simulink library "neural"  (R2016b)
settings: Solver=ode45  StartTime=0.0  StopTime=10.0  RelTol=1e-3
undefined symbols (not defined in the file): sfunxy2
libraries: simulink x2
(part 2 of 2)

== system neural/Transfer Functions/elliotsig ==
  n : Inport
  Abs : Abs
  Divide : Product  Inputs=*/
  Sum : Sum  SaturateOnIntegerOverflow=on  InputSameDT=on  OutDataTypeStr=Inherit: Same as first input
  one : Constant
  a : Outport  InitialOutput=0
  wires:
  Sum/1 -> Divide/2
  Divide/1 -> a/1
  Abs/1 -> Sum/1
  n/1 -> Divide/1, Abs/1
  one/1 -> Sum/2

== system neural/Transfer Functions/hardlim ==
  n : Inport
  Constant : Constant
  Constant1 : Constant  Value=0
  Switch : Switch
  a : Outport  InitialOutput=0
  wires:
  Switch/1 -> a/1
  n/1 -> Switch/2
  Constant1/1 -> Switch/3
  Constant/1 -> Switch/1

== system neural/Transfer Functions/hardlims ==
  n : Inport
  Constant : Constant
  Constant1 : Constant  Value=-1
  Switch : Switch
  a : Outport  InitialOutput=0
  wires:
  Switch/1 -> a/1
  n/1 -> Switch/2
  Constant1/1 -> Switch/3
  Constant/1 -> Switch/1

== system neural/Transfer Functions/logsig ==
  n : Inport
  Exp : Math  SaturateOnIntegerOverflow=on
  Gain : Gain  Gain=-1  SaturateOnIntegerOverflow=on  OutDataTypeStr=Inherit: Same as input  ParamDataTypeStr=Inherit: Same as input
  Reciprocal : Math  Operator=reciprocal  SaturateOnIntegerOverflow=on
  Sum : Sum  SaturateOnIntegerOverflow=on  InputSameDT=on  OutDataTypeStr=Inherit: Same as first input
  one : Constant
  a : Outport  InitialOutput=0
  wires:
  Reciprocal/1 -> a/1
  Sum/1 -> Reciprocal/1
  one/1 -> Sum/2
  Exp/1 -> Sum/1
  Gain/1 -> Exp/1
  n/1 -> Gain/1

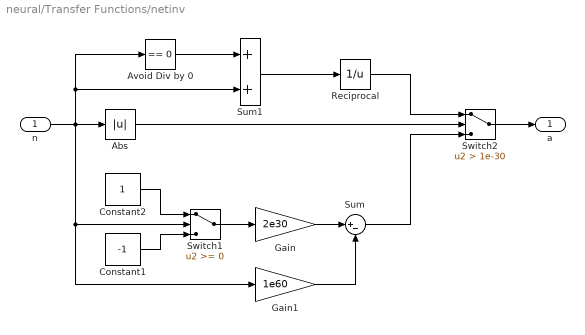
== system neural/Transfer Functions/netinv ==
  n : Inport
  Abs : Abs
  Avoid Div by 0 : simulink/Logic and Bit Operations/Compare To Constant  relop===  const=0  OutDataTypeStr=uint8
  Constant1 : Constant  Value=-1
  Constant2 : Constant
  Gain : Gain  Gain=2e30
  Gain1 : Gain  Gain=1e60
  Reciprocal : Math  Operator=reciprocal  SaturateOnIntegerOverflow=on
  Sum : Sum  Inputs=|+-
  Sum1 : Sum
  Switch1 : Switch
  Switch2 : Switch  Criteria=u2 > Threshold  Threshold=1e-30
  a : Outport  InitialOutput=0
  wires:
  n/1 -> Abs/1, Gain1/1, Switch1/2, Avoid Div by 0/1, Sum1/2
  Abs/1 -> Switch2/2
  Gain/1 -> Sum/1
  Gain1/1 -> Sum/2
  Sum/1 -> Switch2/3
  Constant1/1 -> Switch1/3
  Constant2/1 -> Switch1/1
  Switch1/1 -> Gain/1
  Switch2/1 -> a/1
  Avoid Div by 0/1 -> Sum1/1
  Sum1/1 -> Reciprocal/1
  Reciprocal/1 -> Switch2/1

== system neural/Transfer Functions/poslin ==
  n : Inport
  Saturation : Saturate  UpperLimit=inf  LowerLimit=0
  a : Outport  InitialOutput=0
  wires:
  n/1 -> Saturation/1
  Saturation/1 -> a/1

== system neural/Transfer Functions/purelin ==
  n : Inport
  a : Outport  InitialOutput=0
  wires:
  n/1 -> a/1

== system neural/Transfer Functions/radbas ==
  n : Inport
  Exp : Math  SaturateOnIntegerOverflow=on
  Gain : Gain  Gain=-1  SaturateOnIntegerOverflow=on  OutDataTypeStr=Inherit: Same as input  ParamDataTypeStr=Inherit: Same as input
  Product : Product  SaturateOnIntegerOverflow=on  RndMeth=Zero  InputSameDT=on  OutDataTypeStr=Inherit: Same as first input
  a : Outport  InitialOutput=0
  wires:
  Exp/1 -> a/1
  Gain/1 -> Exp/1
  Product/1 -> Gain/1
  n/1 -> Product/2, Product/1

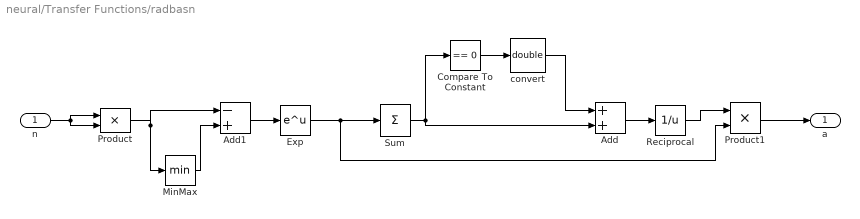
== system neural/Transfer Functions/radbasn ==
  n : Inport
  Add : Sum
  Add1 : Sum  Inputs=-+
  Compare To Constant : simulink/Logic and Bit Operations/Compare To Constant  relop===  const=0  OutDataTypeStr=uint8
  Exp : Math  SaturateOnIntegerOverflow=on
  MinMax : MinMax
  Product : Product  SaturateOnIntegerOverflow=on  RndMeth=Zero  InputSameDT=on  OutDataTypeStr=Inherit: Same as first input
  Product1 : Product  SaturateOnIntegerOverflow=on  RndMeth=Zero  InputSameDT=on  OutDataTypeStr=Inherit: Same as first input
  Reciprocal : Math  Operator=reciprocal  SaturateOnIntegerOverflow=on
  Sum : Sum  Inputs=+  SaturateOnIntegerOverflow=on  InputSameDT=on  OutDataTypeStr=Inherit: Same as first input
  convert : DataTypeConversion  OutDataTypeStr=double
  a : Outport  InitialOutput=0
  wires:
  n/1 -> Product/1, Product/2
  Product/1 -> MinMax/1, Add1/1
  Add1/1 -> Exp/1
  Sum/1 -> Compare To Constant/1, Add/2
  Product1/1 -> a/1
  Reciprocal/1 -> Product1/1
  Exp/1 -> Sum/1, Product1/2
  Compare To Constant/1 -> convert/1
  Add/1 -> Reciprocal/1
  convert/1 -> Add/1
  MinMax/1 -> Add1/2

== system neural/Transfer Functions/satlin ==
  n : Inport
  Saturation : Saturate  UpperLimit=1  LowerLimit=0
  a : Outport  InitialOutput=0
  wires:
  n/1 -> Saturation/1
  Saturation/1 -> a/1

== system neural/Transfer Functions/satlins ==
  n : Inport
  Saturation : Saturate  UpperLimit=1  LowerLimit=-1
  a : Outport  InitialOutput=0
  wires:
  n/1 -> Saturation/1
  Saturation/1 -> a/1

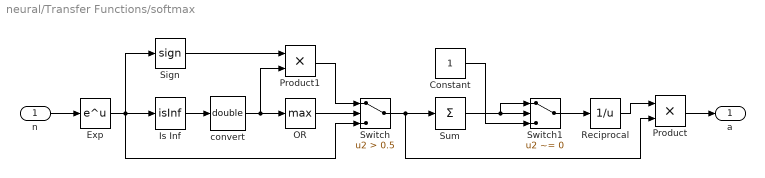
== system neural/Transfer Functions/softmax ==
  n : Inport
  Constant : Constant
  Exp : Math  SaturateOnIntegerOverflow=on
  Is Inf : RelationalOperator  Operator=isInf  OutDataTypeStr=fixdt(1,16)  RndMeth=Nearest
  OR : MinMax  Function=max
  Product : Product  SaturateOnIntegerOverflow=on  RndMeth=Zero  InputSameDT=on  OutDataTypeStr=Inherit: Same as first input
  Product1 : Product  SaturateOnIntegerOverflow=on  RndMeth=Zero  InputSameDT=on  OutDataTypeStr=Inherit: Same as first input
  Reciprocal : Math  Operator=reciprocal  SaturateOnIntegerOverflow=on
  Sign : Signum
  Sum : Sum  Inputs=+  SaturateOnIntegerOverflow=on  InputSameDT=on  OutDataTypeStr=Inherit: Same as first input
  Switch : Switch  Criteria=u2 > Threshold  Threshold=0.5
  Switch1 : Switch  Criteria=u2 ~= 0  Threshold=0.5
  convert : DataTypeConversion  OutDataTypeStr=double
  a : Outport  InitialOutput=0
  wires:
  Product/1 -> a/1
  n/1 -> Exp/1
  Is Inf/1 -> convert/1
  convert/1 -> OR/1, Product1/2
  Switch/1 -> Sum/1, Product/2
  OR/1 -> Switch/2
  Exp/1 -> Switch/3, Sign/1, Is Inf/1
  Sign/1 -> Product1/1
  Product1/1 -> Switch/1
  Switch1/1 -> Reciprocal/1
  Reciprocal/1 -> Product/1
  Sum/1 -> Switch1/2, Switch1/1
  Constant/1 -> Switch1/3

== system neural/Transfer Functions/tansig ==
  n : Inport
  Exp : Math  SaturateOnIntegerOverflow=on
  Gain : Gain  Gain=-2  SaturateOnIntegerOverflow=on  OutDataTypeStr=Inherit: Same as input  ParamDataTypeStr=Inherit: Same as input
  Gain1 : Gain  Gain=2  SaturateOnIntegerOverflow=on  OutDataTypeStr=Inherit: Same as input  ParamDataTypeStr=Inherit: Same as input
  Reciprocal : Math  Operator=reciprocal  SaturateOnIntegerOverflow=on
  Sum : Sum  SaturateOnIntegerOverflow=on  InputSameDT=on  OutDataTypeStr=Inherit: Same as first input
  Sum1 : Sum  Inputs=+-  SaturateOnIntegerOverflow=on  InputSameDT=on  OutDataTypeStr=Inherit: Same as first input
  one : Constant
  one1 : Constant
  a : Outport  InitialOutput=0
  wires:
  Sum1/1 -> a/1
  one1/1 -> Sum1/2
  Gain1/1 -> Sum1/1
  Reciprocal/1 -> Gain1/1
  Sum/1 -> Reciprocal/1
  one/1 -> Sum/2
  Exp/1 -> Sum/1
  Gain/1 -> Exp/1
  n/1 -> Gain/1

== system neural/Transfer Functions/tribas ==
  In1 : Inport
  Abs : Abs  SaturateOnIntegerOverflow=on
  MinMax : MinMax  Function=max  Inputs=2  SaturateOnIntegerOverflow=on  InputSameDT=on
  Sum : Sum  Inputs=+-  SaturateOnIntegerOverflow=on  InputSameDT=on  OutDataTypeStr=Inherit: Same as first input
  one : Constant
  zero : Constant  Value=0
  Out1 : Outport  InitialOutput=0
  wires:
  one/1 -> Sum/1
  In1/1 -> Abs/1
  Abs/1 -> Sum/2
  Sum/1 -> MinMax/1
  zero/1 -> MinMax/2
  MinMax/1 -> Out1/1

== system neural/Weight Functions/dist ==
  w : Inport
  p : Inport  Port=2
  Diff : Sum  Inputs=+-  SaturateOnIntegerOverflow=on  InputSameDT=on  OutDataTypeStr=Inherit: Same as first input
  Product : Product  SaturateOnIntegerOverflow=on  RndMeth=Zero  InputSameDT=on  OutDataTypeStr=Inherit: Same as first input
  Sqrt : Math  Operator=sqrt  SaturateOnIntegerOverflow=on
  Sum : Sum  Inputs=1  SaturateOnIntegerOverflow=on  InputSameDT=on  OutDataTypeStr=Inherit: Same as first input
  z : Outport  InitialOutput=0
  wires:
  Sqrt/1 -> z/1
  Sum/1 -> Sqrt/1
  Product/1 -> Sum/1
  Diff/1 -> Product/2, Product/1
  p/1 -> Diff/2
  w/1 -> Diff/1

== system neural/Weight Functions/dotprod ==
  In1 : Inport
  In2 : Inport  Port=2
  Dot Product : DotProduct  InputSameDT=on  OutDataTypeStr=Inherit: Inherit via internal rule
  Out1 : Outport
  wires:
  In1/1 -> Dot Product/1
  In2/1 -> Dot Product/2
  Dot Product/1 -> Out1/1

== system neural/Weight Functions/negdist ==
  w : Inport
  p : Inport  Port=2
  Diff : Sum  Inputs=+-  SaturateOnIntegerOverflow=on  InputSameDT=on  OutDataTypeStr=Inherit: Same as first input
  Gain : Gain  Gain=-1  SaturateOnIntegerOverflow=on  OutDataTypeStr=Inherit: Same as input  ParamDataTypeStr=Inherit: Same as input
  Product : Product  SaturateOnIntegerOverflow=on  RndMeth=Zero  InputSameDT=on  OutDataTypeStr=Inherit: Same as first input
  Sqrt : Math  Operator=sqrt  SaturateOnIntegerOverflow=on
  Sum : Sum  Inputs=1  SaturateOnIntegerOverflow=on  InputSameDT=on  OutDataTypeStr=Inherit: Same as first input
  z : Outport  InitialOutput=0
  wires:
  Gain/1 -> z/1
  Sqrt/1 -> Gain/1
  Sum/1 -> Sqrt/1
  Product/1 -> Sum/1
  Diff/1 -> Product/2, Product/1
  p/1 -> Diff/2
  w/1 -> Diff/1

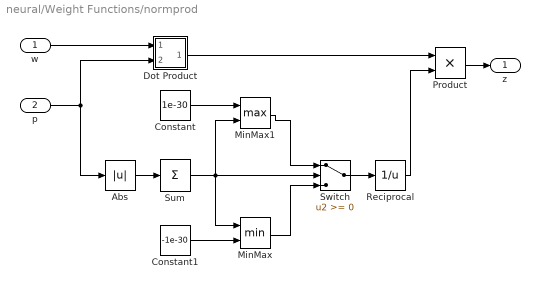
== system neural/Weight Functions/normprod ==
  w : Inport
  p : Inport  Port=2
  Abs : Abs
  Constant : Constant  Value=1e-30
  Constant1 : Constant  Value=-1e-30
  Dot Product : Subsystem  mask(Dot Product){}
      mask help:
      | Inner (dot) product.
      | y=sum(u1.*u2)
      mask init:
      | t=(0:.1:2*pi)';
      | x=cos(t);
      | y=sin(t);
      mask Help: Computes the inner (dot) product of the inputs: sum(u1.*u2).  The inputs are vectors of the same length. Output is a scalar.
      mask Display: plot(0,0,1,1,x*[0.025 0.07]+0.5,y*[0.025 0.07]+0.5)
  MinMax : MinMax  Inputs=2
  MinMax1 : MinMax  Function=max  Inputs=2
  Product : Product  SaturateOnIntegerOverflow=on  RndMeth=Zero  InputSameDT=on  OutDataTypeStr=Inherit: Same as first input
  Reciprocal : Math  Operator=reciprocal  SaturateOnIntegerOverflow=on
  Sum : Sum  Inputs=1  SaturateOnIntegerOverflow=on  InputSameDT=on  OutDataTypeStr=Inherit: Same as first input
  Switch : Switch
  z : Outport  InitialOutput=0
  wires:
  Product/1 -> z/1
  Dot Product/1(out_1) -> Product/1
  p/1 -> Dot Product/2(in_2), Abs/1
  w/1 -> Dot Product/1(in_1)
  Reciprocal/1 -> Product/2
  Sum/1 -> MinMax/1, MinMax1/2, Switch/2
  Constant/1 -> MinMax1/1
  Constant1/1 -> MinMax/2
  MinMax/1 -> Switch/3
  MinMax1/1 -> Switch/1
  Switch/1 -> Reciprocal/1
  Abs/1 -> Sum/1

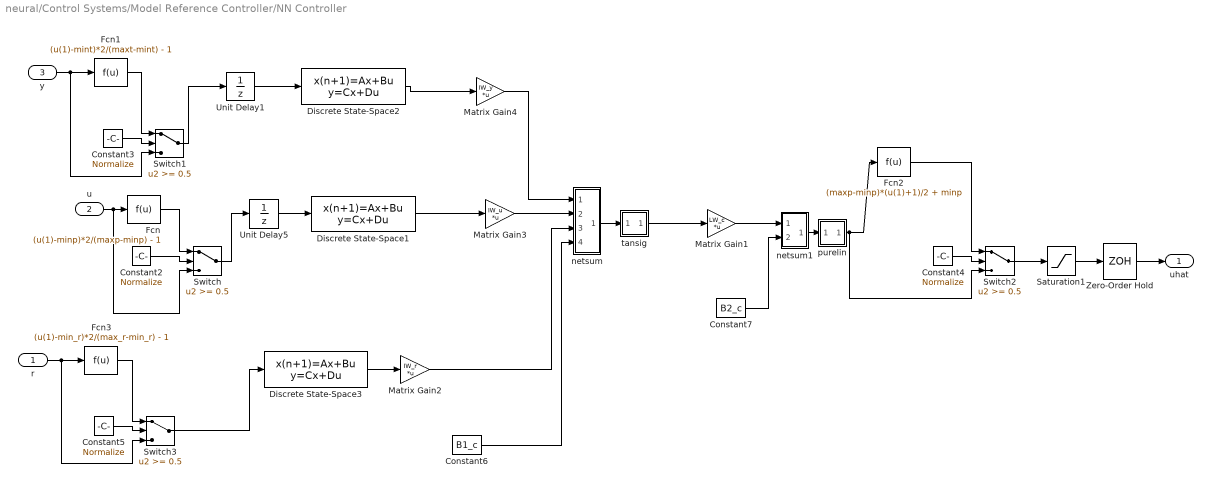
== system neural/Control Systems/Model Reference Controller/NN Controller ==
  r : Inport
  u : Inport  Port=2
  y : Inport  Port=3
  Constant{2..5} (4 alike) : Constant  Value=Normalize
  Constant6 : Constant  Value=B1_c
  Constant7 : Constant  Value=B2_c
  Discrete State-Space1 : DiscreteStateSpace  A=[zeros(1,max([Nic-1 1]));eye(Nic-2,Nic-1)]  B=eye(max([Nic-1 1]),1)  C=[zeros(1,max([Nic-1 1]));eye(Nic-1,Nic-1)]  D=eye(Nic,1)  SampleTime=Ts
  Discrete State-Space2 : DiscreteStateSpace  A=[zeros(1,max([Njc-1 1]));eye(Njc-2,Njc-1)]  B=eye(max([Njc-1 1]),1)  C=[zeros(1,max([Njc-1 1]));eye(Njc-1,Njc-1)]  D=eye(Njc,1)  SampleTime=Ts
  Discrete State-Space3 : DiscreteStateSpace  A=[zeros(1,max([Nrc-1 1]));eye(Nrc-2,Nrc-1)]  B=eye(max([Nrc-1 1]),1)  C=[zeros(1,max([Nrc-1 1]));eye(Nrc-1,Nrc-1)]  D=eye(Nrc,1)  SampleTime=Ts
  Fcn : Fcn  Expr=(u(1)-minp)*2/(maxp-minp) - 1
  Fcn1 : Fcn  Expr=(u(1)-mint)*2/(maxt-mint) - 1
  Fcn2 : Fcn  Expr=(maxp-minp)*(u(1)+1)/2 + minp
  Fcn3 : Fcn  Expr=(u(1)-min_r)*2/(max_r-min_r) - 1
  Matrix Gain1 : Gain  Gain=LW_c  Multiplication=Matrix(K*u)  SaturateOnIntegerOverflow=on  OutDataTypeStr=Inherit: Same as input  ParamDataTypeStr=Inherit: Same as input
  Matrix Gain2 : Gain  Gain=IW_r  Multiplication=Matrix(K*u)  SaturateOnIntegerOverflow=on  OutDataTypeStr=Inherit: Same as input  ParamDataTypeStr=Inherit: Same as input
  Matrix Gain3 : Gain  Gain=IW_u  Multiplication=Matrix(K*u)  SaturateOnIntegerOverflow=on  OutDataTypeStr=Inherit: Same as input  ParamDataTypeStr=Inherit: Same as input
  Matrix Gain4 : Gain  Gain=IW_y  Multiplication=Matrix(K*u)  SaturateOnIntegerOverflow=on  OutDataTypeStr=Inherit: Same as input  ParamDataTypeStr=Inherit: Same as input
  Saturation1 : Saturate  UpperLimit=max_i  LowerLimit=min_i
  Switch{,1..3} (4 alike) : Switch  Threshold=0.5  SaturateOnIntegerOverflow=on  InputSameDT=on
  Unit Delay1 : UnitDelay  SampleTime=Ts
  Unit Delay5 : UnitDelay  SampleTime=Ts
  Zero-Order Hold : ZeroOrderHold  SampleTime=Ts
  netsum : Subsystem
      mask Display: disp('+')
  netsum1 : Subsystem
      mask Display: disp('+')
  purelin : Subsystem
      mask Display: plot([-1 1],[0 0],[-1 1],[-1 1])
  tansig : Subsystem
      mask Display: plot([-1 1],[0 0],[-1 -.9 -.8 -.7 -.6 -.5 -.4 -.3 -.2 -.1 0 .1 .2 .3 .4 .5 .6 .7 .8 .9 1],2./(1+exp(-8*[-1 -.9 -.8 -.7 -.6 -.5 -.4 -.3 -.2 -.1 0 .1 .2 .3 .4 .5 .6 .7 .8 .9 1]))-1)
  uhat : Outport
  wires:
  Fcn2/1 -> Switch2/1
  Fcn/1 -> Switch/1
  Discrete State-Space1/1 -> Matrix Gain3/1
  tansig/1(a) -> Matrix Gain1/1
  Discrete State-Space2/1 -> Matrix Gain4/1
  Switch3/1 -> Discrete State-Space3/1
  Unit Delay1/1 -> Discrete State-Space2/1
  Unit Delay5/1 -> Discrete State-Space1/1
  Saturation1/1 -> Zero-Order Hold/1
  Zero-Order Hold/1 -> uhat/1
  Discrete State-Space3/1 -> Matrix Gain2/1
  Constant7/1 -> netsum1/2(In2)
  Switch2/1 -> Saturation1/1
  purelin/1(a) -> Fcn2/1, Switch2/3
  Constant4/1 -> Switch2/2
  Matrix Gain1/1 -> netsum1/1(In1)
  netsum1/1(Out1) -> purelin/1(n)
  Matrix Gain2/1 -> netsum/3(In3)
  netsum/1(Out1) -> tansig/1(n)
  r/1 -> Switch3/3, Fcn3/1
  Fcn3/1 -> Switch3/1
  Constant5/1 -> Switch3/2
  y/1 -> Switch1/3, Fcn1/1
  Fcn1/1 -> Switch1/1
  Switch1/1 -> Unit Delay1/1
  Constant3/1 -> Switch1/2
  Constant2/1 -> Switch/2
  u/1 -> Fcn/1, Switch/3
  Switch/1 -> Unit Delay5/1
  Constant6/1 -> netsum/4(In4)
  Matrix Gain3/1 -> netsum/2(In2)
  Matrix Gain4/1 -> netsum/1(In1)

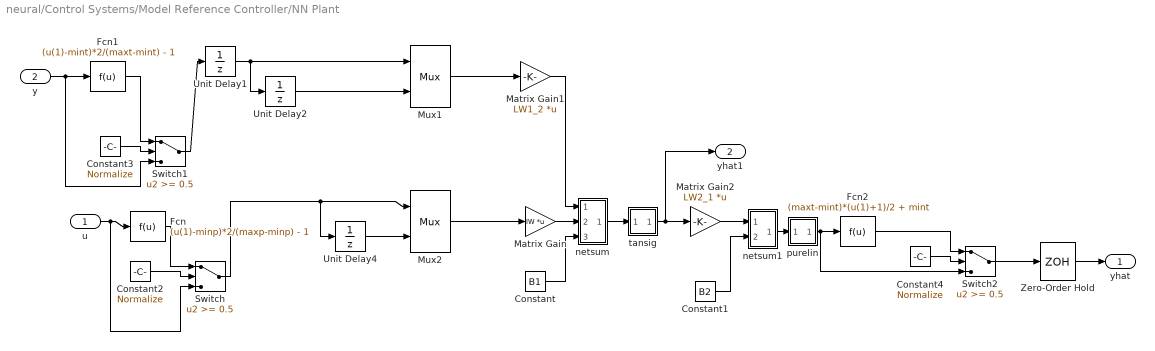
== system neural/Control Systems/Model Reference Controller/NN Plant ==
  u : Inport
  y : Inport  Port=2
  Constant : Constant  Value=B1
  Constant1 : Constant  Value=B2
  Constant2 : Constant  Value=Normalize
  Constant3 : Constant  Value=Normalize
  Constant4 : Constant  Value=Normalize
  Fcn : Fcn  Expr=(u(1)-minp)*2/(maxp-minp) - 1
  Fcn1 : Fcn  Expr=(u(1)-mint)*2/(maxt-mint) - 1
  Fcn2 : Fcn  Expr=(maxt-mint)*(u(1)+1)/2 + mint
  Matrix Gain : Gain  Gain=IW  Multiplication=Matrix(K*u)  SaturateOnIntegerOverflow=on  OutDataTypeStr=Inherit: Same as input  ParamDataTypeStr=Inherit: Same as input
  Matrix Gain1 : Gain  Gain=LW1_2  Multiplication=Matrix(K*u)  SaturateOnIntegerOverflow=on  OutDataTypeStr=Inherit: Same as input  ParamDataTypeStr=Inherit: Same as input
  Matrix Gain2 : Gain  Gain=LW2_1  Multiplication=Matrix(K*u)  SaturateOnIntegerOverflow=on  OutDataTypeStr=Inherit: Same as input  ParamDataTypeStr=Inherit: Same as input
  Mux1 : Mux  Inputs=2
      settings: DisplayOption=signals
  Mux2 : Mux  Inputs=2
      settings: DisplayOption=signals
  Switch : Switch  Threshold=0.5  SaturateOnIntegerOverflow=on  InputSameDT=on
  Switch1 : Switch  Threshold=0.5  SaturateOnIntegerOverflow=on  InputSameDT=on
  Switch2 : Switch  Threshold=0.5  SaturateOnIntegerOverflow=on  InputSameDT=on
  Unit Delay1 : UnitDelay  SampleTime=Ts
  Unit Delay2 : UnitDelay  SampleTime=Ts
  Unit Delay4 : UnitDelay  SampleTime=Ts
  Zero-Order Hold : ZeroOrderHold  SampleTime=Ts
  netsum : Subsystem
      mask Display: disp('+')
  netsum1 : Subsystem
      mask Display: disp('+')
  purelin : Subsystem
      mask Display: plot([-1 1],[0 0],[-1 1],[-1 1])
  tansig : Subsystem
      mask Display: plot([-1 1],[0 0],[-1 -.9 -.8 -.7 -.6 -.5 -.4 -.3 -.2 -.1 0 .1 .2 .3 .4 .5 .6 .7 .8 .9 1],2./(1+exp(-8*[-1 -.9 -.8 -.7 -.6 -.5 -.4 -.3 -.2 -.1 0 .1 .2 .3 .4 .5 .6 .7 .8 .9 1]))-1)
  yhat : Outport
  yhat1 : Outport  Port=2
  wires:
  Switch2/1 -> Zero-Order Hold/1
  Zero-Order Hold/1 -> yhat/1
  Switch/1 -> Unit Delay4/1, Mux2/1
  Unit Delay4/1 -> Mux2/2
  Unit Delay2/1 -> Mux1/2
  Unit Delay1/1 -> Unit Delay2/1, Mux1/1
  y/1 -> Switch1/3, Fcn1/1
  Fcn1/1 -> Switch1/1
  Switch1/1 -> Unit Delay1/1
  Constant3/1 -> Switch1/2
  Mux1/1 -> Matrix Gain1/1
  Constant2/1 -> Switch/2
  u/1 -> Switch/3, Fcn/1
  Fcn/1 -> Switch/1
  Mux2/1 -> Matrix Gain/1
  purelin/1(a) -> Switch2/3, Fcn2/1
  Fcn2/1 -> Switch2/1
  Constant4/1 -> Switch2/2
  tansig/1(a) -> yhat1/1, Matrix Gain2/1
  Matrix Gain/1 -> netsum/2(In2)
  Matrix Gain1/1 -> netsum/1(In1)
  Constant/1 -> netsum/3(In3)
  netsum/1(Out1) -> tansig/1(n)
  Matrix Gain2/1 -> netsum1/1(In1)
  Constant1/1 -> netsum1/2(In2)
  netsum1/1(Out1) -> purelin/1(n)

== system neural/Control Systems/NARMA-L2 Controller/netsum ==
  In1 : Inport
  In2 : Inport  Port=2
  netsum : Sum  Inputs=2  SaturateOnIntegerOverflow=on  InputSameDT=on  OutDataTypeStr=Inherit: Same as first input
  Out1 : Outport
  wires:
  netsum/1 -> Out1/1
  In2/1 -> netsum/2
  In1/1 -> netsum/1

== system neural/Control Systems/NARMA-L2 Controller/netsum1 ==
  In1 : Inport
  In2 : Inport  Port=2
  netsum1 : Sum  Inputs=2  SaturateOnIntegerOverflow=on  InputSameDT=on  OutDataTypeStr=Inherit: Same as first input
  Out1 : Outport
  wires:
  netsum1/1 -> Out1/1
  In2/1 -> netsum1/2
  In1/1 -> netsum1/1

== system neural/Control Systems/NARMA-L2 Controller/netsum2 ==
  In1 : Inport
  In2 : Inport  Port=2
  netsum : Sum  Inputs=2  SaturateOnIntegerOverflow=on  InputSameDT=on  OutDataTypeStr=Inherit: Same as first input
  Out1 : Outport
  wires:
  netsum/1 -> Out1/1
  In2/1 -> netsum/2
  In1/1 -> netsum/1

== system neural/Control Systems/NARMA-L2 Controller/netsum3 ==
  In1 : Inport
  In2 : Inport  Port=2
  netsum1 : Sum  Inputs=2  SaturateOnIntegerOverflow=on  InputSameDT=on  OutDataTypeStr=Inherit: Same as first input
  Out1 : Outport
  wires:
  netsum1/1 -> Out1/1
  In2/1 -> netsum1/2
  In1/1 -> netsum1/1

== system neural/Control Systems/NARMA-L2 Controller/purelin ==
  n : Inport
  a : Outport
  wires:
  n/1 -> a/1

== system neural/Control Systems/NARMA-L2 Controller/purelin1 ==
  n : Inport
  a : Outport
  wires:
  n/1 -> a/1

== system neural/Control Systems/NARMA-L2 Controller/tansig ==
  n : Inport
  Exp : Math  SaturateOnIntegerOverflow=on
  Gain : Gain  Gain=-2  SaturateOnIntegerOverflow=on  OutDataTypeStr=Inherit: Same as input  ParamDataTypeStr=Inherit: Same as input
  Gain1 : Gain  Gain=2  SaturateOnIntegerOverflow=on  OutDataTypeStr=Inherit: Same as input  ParamDataTypeStr=Inherit: Same as input
  Reciprocal : Math  Operator=reciprocal  SaturateOnIntegerOverflow=on
  Sum : Sum  SaturateOnIntegerOverflow=on  InputSameDT=on  OutDataTypeStr=Inherit: Same as first input
  Sum1 : Sum  Inputs=+-  SaturateOnIntegerOverflow=on  InputSameDT=on  OutDataTypeStr=Inherit: Same as first input
  one : Constant
  one1 : Constant
  a : Outport
  wires:
  Sum1/1 -> a/1
  one1/1 -> Sum1/2
  Gain1/1 -> Sum1/1
  Reciprocal/1 -> Gain1/1
  Sum/1 -> Reciprocal/1
  one/1 -> Sum/2
  Exp/1 -> Sum/1
  Gain/1 -> Exp/1
  n/1 -> Gain/1

== system neural/Control Systems/NARMA-L2 Controller/tansig1 ==
  n : Inport
  Exp : Math  SaturateOnIntegerOverflow=on
  Gain : Gain  Gain=-2  SaturateOnIntegerOverflow=on  OutDataTypeStr=Inherit: Same as input  ParamDataTypeStr=Inherit: Same as input
  Gain1 : Gain  Gain=2  SaturateOnIntegerOverflow=on  OutDataTypeStr=Inherit: Same as input  ParamDataTypeStr=Inherit: Same as input
  Reciprocal : Math  Operator=reciprocal  SaturateOnIntegerOverflow=on
  Sum : Sum  SaturateOnIntegerOverflow=on  InputSameDT=on  OutDataTypeStr=Inherit: Same as first input
  Sum1 : Sum  Inputs=+-  SaturateOnIntegerOverflow=on  InputSameDT=on  OutDataTypeStr=Inherit: Same as first input
  one : Constant
  one1 : Constant
  a : Outport
  wires:
  Sum1/1 -> a/1
  one1/1 -> Sum1/2
  Gain1/1 -> Sum1/1
  Reciprocal/1 -> Gain1/1
  Sum/1 -> Reciprocal/1
  one/1 -> Sum/2
  Exp/1 -> Sum/1
  Gain/1 -> Exp/1
  n/1 -> Gain/1

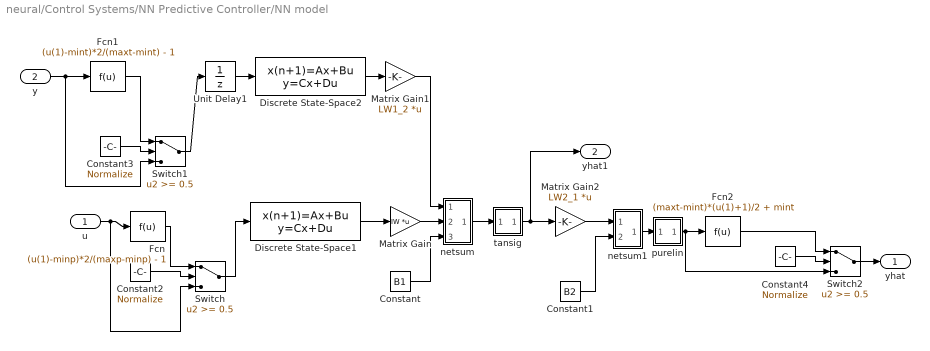
== system neural/Control Systems/NN Predictive Controller/NN model ==
  u : Inport
  y : Inport  Port=2
  Constant : Constant  Value=B1
  Constant1 : Constant  Value=B2
  Constant2 : Constant  Value=Normalize
  Constant3 : Constant  Value=Normalize
  Constant4 : Constant  Value=Normalize
  Discrete State-Space1 : DiscreteStateSpace  A=[0 zeros(1,Ni-2);eye(Ni-2,Ni-1)]  B=[zeros(double(Ni==1));eye(Ni-1,1)]  C=[0 zeros(1,Ni-2);eye(Ni-1,Ni-1)]  D=eye(Ni,1)  SampleTime=Ts
  Discrete State-Space2 : DiscreteStateSpace  A=[0 zeros(1,Nj-2);eye(Nj-2,Nj-1)]  B=[zeros(double(Nj==1));eye(Nj-1,1)]  C=[0 zeros(1,Nj-2);eye(Nj-1,Nj-1)]  D=eye(Nj,1)  SampleTime=Ts
  Fcn : Fcn  Expr=(u(1)-minp)*2/(maxp-minp) - 1
  Fcn1 : Fcn  Expr=(u(1)-mint)*2/(maxt-mint) - 1
  Fcn2 : Fcn  Expr=(maxt-mint)*(u(1)+1)/2 + mint
  Matrix Gain : Gain  Gain=IW  Multiplication=Matrix(K*u)  SaturateOnIntegerOverflow=on  OutDataTypeStr=Inherit: Same as input  ParamDataTypeStr=Inherit: Same as input
  Matrix Gain1 : Gain  Gain=LW1_2  Multiplication=Matrix(K*u)  SaturateOnIntegerOverflow=on  OutDataTypeStr=Inherit: Same as input  ParamDataTypeStr=Inherit: Same as input
  Matrix Gain2 : Gain  Gain=LW2_1  Multiplication=Matrix(K*u)  SaturateOnIntegerOverflow=on  OutDataTypeStr=Inherit: Same as input  ParamDataTypeStr=Inherit: Same as input
  Switch : Switch  Threshold=0.5  SaturateOnIntegerOverflow=on  InputSameDT=on
  Switch1 : Switch  Threshold=0.5  SaturateOnIntegerOverflow=on  InputSameDT=on
  Switch2 : Switch  Threshold=0.5  SaturateOnIntegerOverflow=on  InputSameDT=on
  Unit Delay1 : UnitDelay  SampleTime=Ts
  netsum : Subsystem
      mask Display: disp('+')
  netsum1 : Subsystem
      mask Display: disp('+')
  purelin : Subsystem
      mask Display: plot([-1 1],[0 0],[-1 1],[-1 1])
  tansig : Subsystem
      mask Display: plot([-1 1],[0 0],[-1 -.9 -.8 -.7 -.6 -.5 -.4 -.3 -.2 -.1 0 .1 .2 .3 .4 .5 .6 .7 .8 .9 1],2./(1+exp(-8*[-1 -.9 -.8 -.7 -.6 -.5 -.4 -.3 -.2 -.1 0 .1 .2 .3 .4 .5 .6 .7 .8 .9 1]))-1)
  yhat : Outport
  yhat1 : Outport  Port=2
  wires:
  netsum1/1(Out1) -> purelin/1(n)
  Constant1/1 -> netsum1/2(In2)
  Matrix Gain2/1 -> netsum1/1(In1)
  netsum/1(Out1) -> tansig/1(n)
  Constant/1 -> netsum/3(In3)
  Matrix Gain1/1 -> netsum/1(In1)
  Matrix Gain/1 -> netsum/2(In2)
  tansig/1(a) -> Matrix Gain2/1, yhat1/1
  Discrete State-Space1/1 -> Matrix Gain/1
  Fcn/1 -> Switch/1
  Switch/1 -> Discrete State-Space1/1
  u/1 -> Fcn/1, Switch/3
  Constant2/1 -> Switch/2
  Discrete State-Space2/1 -> Matrix Gain1/1
  Unit Delay1/1 -> Discrete State-Space2/1
  Constant3/1 -> Switch1/2
  Switch1/1 -> Unit Delay1/1
  Fcn1/1 -> Switch1/1
  y/1 -> Fcn1/1, Switch1/3
  Constant4/1 -> Switch2/2
  Switch2/1 -> yhat/1
  Fcn2/1 -> Switch2/1
  purelin/1(a) -> Fcn2/1, Switch2/3

== system neural/Weight Functions/normprod/Dot Product ==
  in_1 : Inport
  in_2 : Inport  Port=2
  Product : Product  SaturateOnIntegerOverflow=on  RndMeth=Zero  InputSameDT=on  OutDataTypeStr=Inherit: Same as first input
  Sum : Sum  Inputs=+  SaturateOnIntegerOverflow=on  InputSameDT=on  OutDataTypeStr=Inherit: Same as first input
  out_1 : Outport  InitialOutput=0
  wires:
  Sum/1 -> out_1/1
  Product/1 -> Sum/1
  in_1/1 -> Product/1
  in_2/1 -> Product/2

== system neural/Control Systems/Model Reference Controller/NN Controller/netsum ==
  In1 : Inport
  In2 : Inport  Port=2
  In3 : Inport  Port=3
  In4 : Inport  Port=4
  netsum : Sum  Inputs=4  SaturateOnIntegerOverflow=on  InputSameDT=on  OutDataTypeStr=Inherit: Same as first input
  Out1 : Outport
  wires:
  In4/1 -> netsum/4
  In3/1 -> netsum/3
  netsum/1 -> Out1/1
  In2/1 -> netsum/2
  In1/1 -> netsum/1

== system neural/Control Systems/Model Reference Controller/NN Controller/netsum1 ==
  In1 : Inport
  In2 : Inport  Port=2
  netsum1 : Sum  Inputs=2  SaturateOnIntegerOverflow=on  InputSameDT=on  OutDataTypeStr=Inherit: Same as first input
  Out1 : Outport
  wires:
  netsum1/1 -> Out1/1
  In2/1 -> netsum1/2
  In1/1 -> netsum1/1

== system neural/Control Systems/Model Reference Controller/NN Controller/purelin ==
  n : Inport
  a : Outport
  wires:
  n/1 -> a/1

== system neural/Control Systems/Model Reference Controller/NN Controller/tansig ==
  n : Inport
  Exp : Math  SaturateOnIntegerOverflow=on
  Gain : Gain  Gain=-2  SaturateOnIntegerOverflow=on  OutDataTypeStr=Inherit: Same as input  ParamDataTypeStr=Inherit: Same as input
  Gain1 : Gain  Gain=2  SaturateOnIntegerOverflow=on  OutDataTypeStr=Inherit: Same as input  ParamDataTypeStr=Inherit: Same as input
  Reciprocal : Math  Operator=reciprocal  SaturateOnIntegerOverflow=on
  Sum : Sum  SaturateOnIntegerOverflow=on  InputSameDT=on  OutDataTypeStr=Inherit: Same as first input
  Sum1 : Sum  Inputs=+-  SaturateOnIntegerOverflow=on  InputSameDT=on  OutDataTypeStr=Inherit: Same as first input
  one : Constant
  one1 : Constant
  a : Outport
  wires:
  Sum1/1 -> a/1
  one1/1 -> Sum1/2
  Gain1/1 -> Sum1/1
  Reciprocal/1 -> Gain1/1
  Sum/1 -> Reciprocal/1
  one/1 -> Sum/2
  Exp/1 -> Sum/1
  Gain/1 -> Exp/1
  n/1 -> Gain/1

== system neural/Control Systems/Model Reference Controller/NN Plant/netsum ==
  In1 : Inport
  In2 : Inport  Port=2
  In3 : Inport  Port=3
  netsum : Sum  Inputs=3  SaturateOnIntegerOverflow=on  InputSameDT=on  OutDataTypeStr=Inherit: Same as first input
  Out1 : Outport
  wires:
  netsum/1 -> Out1/1
  In3/1 -> netsum/3
  In2/1 -> netsum/2
  In1/1 -> netsum/1

== system neural/Control Systems/Model Reference Controller/NN Plant/netsum1 ==
  In1 : Inport
  In2 : Inport  Port=2
  netsum1 : Sum  Inputs=2  SaturateOnIntegerOverflow=on  InputSameDT=on  OutDataTypeStr=Inherit: Same as first input
  Out1 : Outport
  wires:
  netsum1/1 -> Out1/1
  In2/1 -> netsum1/2
  In1/1 -> netsum1/1

== system neural/Control Systems/Model Reference Controller/NN Plant/purelin ==
  n : Inport
  a : Outport
  wires:
  n/1 -> a/1

== system neural/Control Systems/Model Reference Controller/NN Plant/tansig ==
  n : Inport
  Exp : Math  SaturateOnIntegerOverflow=on
  Gain : Gain  Gain=-2  SaturateOnIntegerOverflow=on  OutDataTypeStr=Inherit: Same as input  ParamDataTypeStr=Inherit: Same as input
  Gain1 : Gain  Gain=2  SaturateOnIntegerOverflow=on  OutDataTypeStr=Inherit: Same as input  ParamDataTypeStr=Inherit: Same as input
  Reciprocal : Math  Operator=reciprocal  SaturateOnIntegerOverflow=on
  Sum : Sum  SaturateOnIntegerOverflow=on  InputSameDT=on  OutDataTypeStr=Inherit: Same as first input
  Sum1 : Sum  Inputs=+-  SaturateOnIntegerOverflow=on  InputSameDT=on  OutDataTypeStr=Inherit: Same as first input
  one : Constant
  one1 : Constant
  a : Outport
  wires:
  Sum1/1 -> a/1
  one1/1 -> Sum1/2
  Gain1/1 -> Sum1/1
  Reciprocal/1 -> Gain1/1
  Sum/1 -> Reciprocal/1
  one/1 -> Sum/2
  Exp/1 -> Sum/1
  Gain/1 -> Exp/1
  n/1 -> Gain/1

== system neural/Control Systems/NN Predictive Controller/NN model/netsum ==
  In1 : Inport
  In2 : Inport  Port=2
  In3 : Inport  Port=3
  netsum : Sum  Inputs=3  SaturateOnIntegerOverflow=on  InputSameDT=on  OutDataTypeStr=Inherit: Same as first input
  Out1 : Outport
  wires:
  In1/1 -> netsum/1
  In2/1 -> netsum/2
  In3/1 -> netsum/3
  netsum/1 -> Out1/1

== system neural/Control Systems/NN Predictive Controller/NN model/netsum1 ==
  In1 : Inport
  In2 : Inport  Port=2
  netsum1 : Sum  Inputs=2  SaturateOnIntegerOverflow=on  InputSameDT=on  OutDataTypeStr=Inherit: Same as first input
  Out1 : Outport
  wires:
  In1/1 -> netsum1/1
  In2/1 -> netsum1/2
  netsum1/1 -> Out1/1

== system neural/Control Systems/NN Predictive Controller/NN model/purelin ==
  n : Inport
  a : Outport
  wires:
  n/1 -> a/1

== system neural/Control Systems/NN Predictive Controller/NN model/tansig ==
  n : Inport
  Exp : Math  SaturateOnIntegerOverflow=on
  Gain : Gain  Gain=-2  SaturateOnIntegerOverflow=on  OutDataTypeStr=Inherit: Same as input  ParamDataTypeStr=Inherit: Same as input
  Gain1 : Gain  Gain=2  SaturateOnIntegerOverflow=on  OutDataTypeStr=Inherit: Same as input  ParamDataTypeStr=Inherit: Same as input
  Reciprocal : Math  Operator=reciprocal  SaturateOnIntegerOverflow=on
  Sum : Sum  SaturateOnIntegerOverflow=on  InputSameDT=on  OutDataTypeStr=Inherit: Same as first input
  Sum1 : Sum  Inputs=+-  SaturateOnIntegerOverflow=on  InputSameDT=on  OutDataTypeStr=Inherit: Same as first input
  one : Constant
  one1 : Constant
  a : Outport
  wires:
  n/1 -> Gain/1
  Gain/1 -> Exp/1
  Exp/1 -> Sum/1
  one/1 -> Sum/2
  Sum/1 -> Reciprocal/1
  Reciprocal/1 -> Gain1/1
  Gain1/1 -> Sum1/1
  one1/1 -> Sum1/2
  Sum1/1 -> a/1
